simulink model "TTS2_EXT"  (R2024b)
settings: Solver=FixedStepAuto  StartTime=0.0  StopTime=inf  FixedStep=0.01  RelTol=1e-3
model workspace (MAT data in the model file):
  amp_f1 = -100
  amp_f10 = 0.5
  amp_f11 = -0.1
  amp_f12 = 1
  amp_f13 = 0.5
  amp_f14 = -20
  amp_f15 = 0.5
  amp_f16 = 0.5
  amp_f17 = 20
  amp_f18 = -30
  amp_f19 = 0.1
  amp_f2 = -20
  amp_f20 = -20
  amp_f21 = 20
  amp_f3 = -30
  amp_f4 = -30
  amp_f5 = -10
  amp_f51 = -10
  amp_f52 = -30
  amp_f53 = -30
  amp_f54 = 20
  amp_f55 = -100
  amp_f6 = -30
  amp_f7 = -30
  amp_f8 = -30
  amp_f9 = 1
  from_f1 = 570
  from_f10 = 5970
  from_f11 = 6570
  from_f12 = 7170
  from_f13 = 7770
  from_f14 = 8370
  from_f15 = 8970
  from_f16 = 9570
  from_f17 = 10170
  from_f18 = 10770
  from_f19 = 11370
  from_f2 = 1170
  from_f20 = 11970
  from_f21 = 12570
  from_f3 = 1770
  from_f4 = 2370
  from_f5 = 2970
  from_f51 = 13170
  from_f52 = 13770
  from_f53 = 14370
  from_f54 = 14970
  from_f55 = 15570
  from_f6 = 3570
  from_f7 = 4170
  from_f8 = 4770
  from_f9 = 5370
libraries: simulink x52, lab310_library x26, opclib x3
(part 3 of 3)

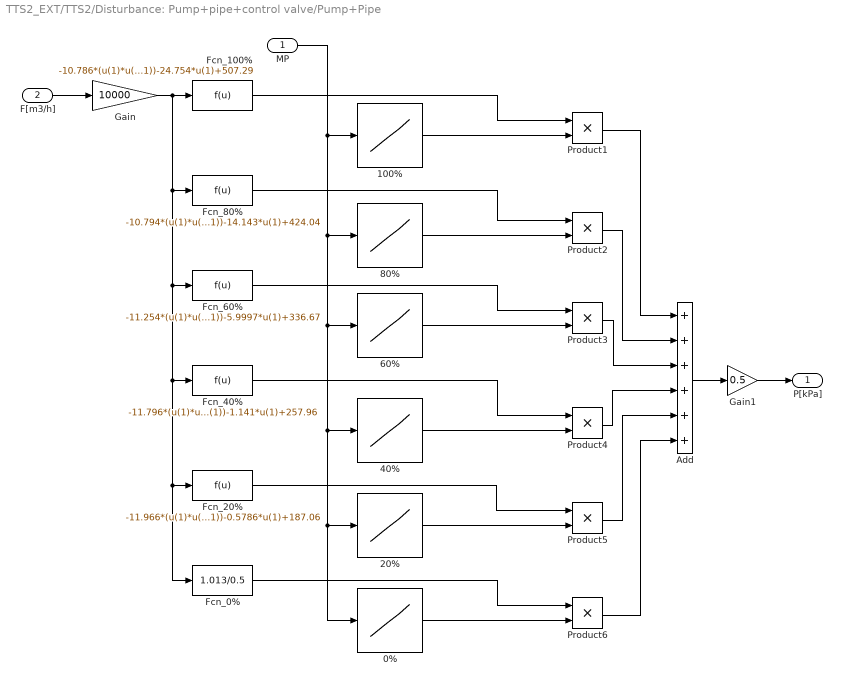
== system TTS2_EXT/TTS2/Disturbance: Pump+pipe+control valve/Pump+Pipe ==
  MP : Inport
  F[m3/h] : Inport  Port=2
  "0% " : Lookup_n-D  NumberOfTableDimensions=1  BreakpointsForDimension1=[0 20 100]  Table=[1 0 0]  InternalRulePriority=Speed  RndMeth=Simplest
  100% : Lookup_n-D  NumberOfTableDimensions=1  BreakpointsForDimension1=[0 80 100]  Table=[0 0 1]  InternalRulePriority=Speed  RndMeth=Simplest
  20% : Lookup_n-D  NumberOfTableDimensions=1  BreakpointsForDimension1=[0 20 40 100]  Table=[0 1 0 0]  InternalRulePriority=Speed  RndMeth=Simplest
  40% : Lookup_n-D  NumberOfTableDimensions=1  BreakpointsForDimension1=[0 20 40 60 100]  Table=[0 0 1 0 0]  InternalRulePriority=Speed  RndMeth=Simplest
  60% : Lookup_n-D  NumberOfTableDimensions=1  BreakpointsForDimension1=[0 40 60 80 100]  Table=[0 0 1 0 0]  InternalRulePriority=Speed  RndMeth=Simplest
  80% : Lookup_n-D  NumberOfTableDimensions=1  BreakpointsForDimension1=[0 60 80 100]  Table=[0 0 1 0]  InternalRulePriority=Speed  RndMeth=Simplest
  Add : Sum  Inputs=6
  Fcn_0% : Fcn  Expr=1.013/0.5
  Fcn_100% : Fcn  Expr=-10.786*(u(1)*u(1))-24.754*u(1)+507.29
  Fcn_20% : Fcn  Expr=-11.966*(u(1)*u(1))-0.5786*u(1)+187.06
  Fcn_40% : Fcn  Expr=-11.796*(u(1)*u(1))-1.141*u(1)+257.96
  Fcn_60% : Fcn  Expr=-11.254*(u(1)*u(1))-5.9997*u(1)+336.67
  Fcn_80% : Fcn  Expr=-10.794*(u(1)*u(1))-14.143*u(1)+424.04
  Gain : Gain  Gain=10000
  Gain1 : Gain  Gain=0.5
  Product{1..6} (6 alike) : Product
  P[kPa] : Outport  VectorParamsAs1DForOutWhenUnconnected=off
  wires:
  F[m3/h]/1 -> Gain/1
  MP/1 -> 80%/1, 40%/1, 20%/1, "0% "/1, 60%/1, 100%/1
  "0% "/1 -> Product6/2
  20%/1 -> Product5/2
  40%/1 -> Product4/2
  60%/1 -> Product3/2
  80%/1 -> Product2/2
  100%/1 -> Product1/2
  Gain/1 -> Fcn_20%/1, Fcn_0%/1, Fcn_40%/1, Fcn_60%/1, Fcn_80%/1, Fcn_100%/1
  Fcn_0%/1 -> Product6/1
  Fcn_20%/1 -> Product5/1
  Fcn_40%/1 -> Product4/1
  Fcn_60%/1 -> Product3/1
  Fcn_80%/1 -> Product2/1
  Fcn_100%/1 -> Product1/1
  Product1/1 -> Add/1
  Product2/1 -> Add/2
  Product3/1 -> Add/3
  Product4/1 -> Add/4
  Product5/1 -> Add/5
  Product6/1 -> Add/6
  Add/1 -> Gain1/1
  Gain1/1 -> P[kPa]/1

== system TTS2_EXT/TTS2/Disturbance: Pump+pipe+control valve/VB ==
  CV[%] : Inport
  P1[kPa] : Inport  Port=2
  P2[kPa] : Inport  Port=3
  Positioner : Subsystem
  Valve : Subsystem
  F[m3/h] : Outport  VectorParamsAs1DForOutWhenUnconnected=off
  wires:
  Valve/1(F[m3/h]) -> F[m3/h]/1
  P1[kPa]/1 -> Valve/2(P1[kPa])
  P2[kPa]/1 -> Valve/3(P2[kPa])
  CV[%]/1 -> Positioner/1(CV[0-100])
  Positioner/1(X[0-1]) -> Valve/1(G[0-1])

== system TTS2_EXT/TTS2/Noise/F1 noise ==
  X : Inport
  Random Number : RandomNumber  Variance=0.006889  Seed=3341  SampleTime=1
  Sum : Sum  Inputs=|++
  X' : Outport  VectorParamsAs1DForOutWhenUnconnected=off
  wires:
  Random Number/1 -> Sum/2
  X/1 -> Sum/1
  Sum/1 -> X'/1

== system TTS2_EXT/TTS2/Noise/F2 noise ==
  X : Inport
  Random Number : RandomNumber  Variance=0.0225  Seed=765756  SampleTime=1
  Sum : Sum  Inputs=|++
  X' : Outport  VectorParamsAs1DForOutWhenUnconnected=off
  wires:
  Random Number/1 -> Sum/2
  X/1 -> Sum/1
  Sum/1 -> X'/1

== system TTS2_EXT/TTS2/Noise/F3 dist ==
  X : Inport
  Random Number : RandomNumber  Variance=0.0225  Seed=756756  SampleTime=1
  Sum : Sum  Inputs=|++
  X' : Outport  VectorParamsAs1DForOutWhenUnconnected=off
  wires:
  Random Number/1 -> Sum/2
  X/1 -> Sum/1
  Sum/1 -> X'/1

== system TTS2_EXT/TTS2/Noise/G noise ==
  X : Inport
  Random Number : RandomNumber  Variance=0.006889  Seed=2312  SampleTime=1
  Sum : Sum  Inputs=|++
  X' : Outport  VectorParamsAs1DForOutWhenUnconnected=off
  wires:
  Random Number/1 -> Sum/2
  X/1 -> Sum/1
  Sum/1 -> X'/1

== system TTS2_EXT/TTS2/Noise/G2 noise ==
  X : Inport
  Random Number : RandomNumber  Variance=0.0225  Seed=75675675  SampleTime=1
  Sum : Sum  Inputs=|++
  X' : Outport  VectorParamsAs1DForOutWhenUnconnected=off
  wires:
  Random Number/1 -> Sum/2
  X/1 -> Sum/1
  Sum/1 -> X'/1

== system TTS2_EXT/TTS2/Noise/L11 noise ==
  X : Inport
  Random Number : RandomNumber  Variance=0.000002777  Seed=4324  SampleTime=1
  Sum : Sum  Inputs=|++
  X' : Outport  VectorParamsAs1DForOutWhenUnconnected=off
  wires:
  Random Number/1 -> Sum/2
  X/1 -> Sum/1
  Sum/1 -> X'/1

== system TTS2_EXT/TTS2/Noise/L12 noise ==
  X : Inport
  Random Number : RandomNumber  Variance=0.00000053777  Seed=432423  SampleTime=1
  Sum : Sum  Inputs=|++
  X' : Outport  VectorParamsAs1DForOutWhenUnconnected=off
  wires:
  Random Number/1 -> Sum/2
  X/1 -> Sum/1
  Sum/1 -> X'/1

== system TTS2_EXT/TTS2/Noise/L21 noise ==
  X : Inport
  Random Number : RandomNumber  Variance=0.000000111111111  Seed=43243423  SampleTime=1
  Sum : Sum  Inputs=|++
  X' : Outport  VectorParamsAs1DForOutWhenUnconnected=off
  wires:
  Random Number/1 -> Sum/2
  X/1 -> Sum/1
  Sum/1 -> X'/1

== system TTS2_EXT/TTS2/Noise/L22 noise ==
  X : Inport
  Random Number : RandomNumber  Variance=0.0000001111111111  Seed=32423  SampleTime=1
  Sum : Sum  Inputs=|++
  X' : Outport  VectorParamsAs1DForOutWhenUnconnected=off
  wires:
  Random Number/1 -> Sum/2
  X/1 -> Sum/1
  Sum/1 -> X'/1

== system TTS2_EXT/TTS2/Noise/L31 noise ==
  X : Inport
  Random Number : RandomNumber  Variance=0.0000017777  Seed=432454  SampleTime=1
  Sum : Sum  Inputs=|++
  X' : Outport  VectorParamsAs1DForOutWhenUnconnected=off
  wires:
  Random Number/1 -> Sum/2
  X/1 -> Sum/1
  Sum/1 -> X'/1

== system TTS2_EXT/TTS2/Noise/L32 noise ==
  X : Inport
  Random Number : RandomNumber  Variance=0.0000006944  Seed=4563565  SampleTime=1
  Sum : Sum  Inputs=|++
  X' : Outport  VectorParamsAs1DForOutWhenUnconnected=off
  wires:
  Random Number/1 -> Sum/2
  X/1 -> Sum/1
  Sum/1 -> X'/1

== system TTS2_EXT/TTS2/Noise/P Dist ==
  X : Inport
  Random Number : RandomNumber  Variance=0.09  Seed=32321  SampleTime=1
  Sum : Sum  Inputs=|++
  X' : Outport  VectorParamsAs1DForOutWhenUnconnected=off
  wires:
  Random Number/1 -> Sum/2
  X/1 -> Sum/1
  Sum/1 -> X'/1

== system TTS2_EXT/TTS2/Noise/dP dist ==
  X : Inport
  Random Number : RandomNumber  Variance=0.09  Seed=756756756  SampleTime=1
  Sum : Sum  Inputs=|++
  X' : Outport  VectorParamsAs1DForOutWhenUnconnected=off
  wires:
  Random Number/1 -> Sum/2
  X/1 -> Sum/1
  Sum/1 -> X'/1

== system TTS2_EXT/TTS2/Noise/f11 fault ==
  X : Inport
  str. : Inport  Port=2
  Add : Sum
  Fcn : Fcn  Expr=u(1)*((u(2)/100)+1)
  Manual Switch : ManualSwitch
  Mux : Mux  Inputs=2
  X' : Outport  VectorParamsAs1DForOutWhenUnconnected=off
  wires:
  Mux/1 -> Fcn/1
  X/1 -> Add/1, Mux/1
  str./1 -> Add/2, Mux/2
  Add/1 -> Manual Switch/1
  Fcn/1 -> Manual Switch/2
  Manual Switch/1 -> X'/1

== system TTS2_EXT/TTS2/Noise/f14 fault ==
  X : Inport
  str. : Inport  Port=2
  Add : Sum
  Fcn : Fcn  Expr=u(1)*((u(2)/100)+1)
  Manual Switch : ManualSwitch  CurrentSetting=0
  Mux : Mux  Inputs=2
  X' : Outport  VectorParamsAs1DForOutWhenUnconnected=off
  wires:
  Mux/1 -> Fcn/1
  X/1 -> Add/1, Mux/1
  str./1 -> Add/2, Mux/2
  Add/1 -> Manual Switch/1
  Fcn/1 -> Manual Switch/2
  Manual Switch/1 -> X'/1

== system TTS2_EXT/TTS2/Noise/f17 fault ==
  X : Inport
  str. : Inport  Port=2
  Add : Sum
  Fcn : Fcn  Expr=u(1)*((u(2)/100)+1)
  Manual Switch : ManualSwitch  CurrentSetting=0
  Mux : Mux  Inputs=2
  X' : Outport  VectorParamsAs1DForOutWhenUnconnected=off
  wires:
  Mux/1 -> Fcn/1
  X/1 -> Add/1, Mux/1
  str./1 -> Add/2, Mux/2
  Add/1 -> Manual Switch/1
  Fcn/1 -> Manual Switch/2
  Manual Switch/1 -> X'/1

== system TTS2_EXT/TTS2/Noise/f18 fault ==
  X : Inport
  str. : Inport  Port=2
  Add : Sum
  Fcn : Fcn  Expr=u(1)*((u(2)/100)+1)
  Manual Switch : ManualSwitch  CurrentSetting=0
  Mux : Mux  Inputs=2
  X' : Outport  VectorParamsAs1DForOutWhenUnconnected=off
  wires:
  Mux/1 -> Fcn/1
  X/1 -> Add/1, Mux/1
  str./1 -> Add/2, Mux/2
  Fcn/1 -> Manual Switch/2
  Manual Switch/1 -> X'/1
  Add/1 -> Manual Switch/1

== system TTS2_EXT/TTS2/Noise/f19 fault ==
  X : Inport
  str. : Inport  Port=2
  Add : Sum
  Fcn : Fcn  Expr=u(1)*((u(2)/100)+1)
  Manual Switch : ManualSwitch
  Mux : Mux  Inputs=2
  X' : Outport  VectorParamsAs1DForOutWhenUnconnected=off
  wires:
  Mux/1 -> Fcn/1
  X/1 -> Add/1, Mux/1
  str./1 -> Add/2, Mux/2
  Add/1 -> Manual Switch/1
  Fcn/1 -> Manual Switch/2
  Manual Switch/1 -> X'/1

== system TTS2_EXT/TTS2/Noise/f20 fault ==
  X : Inport
  str. : Inport  Port=2
  Add : Sum
  Fcn : Fcn  Expr=u(1)*((u(2)/100)+1)
  Manual Switch : ManualSwitch  CurrentSetting=0
  Mux : Mux  Inputs=2
  X' : Outport  VectorParamsAs1DForOutWhenUnconnected=off
  wires:
  Mux/1 -> Fcn/1
  X/1 -> Add/1, Mux/1
  str./1 -> Add/2, Mux/2
  Add/1 -> Manual Switch/1
  Fcn/1 -> Manual Switch/2
  Manual Switch/1 -> X'/1

== system TTS2_EXT/TTS2/Noise/f21 fault ==
  X : Inport
  str. : Inport  Port=2
  Add : Sum
  Fcn : Fcn  Expr=u(1)*((u(2)/100)+1)
  Manual Switch : ManualSwitch  CurrentSetting=0
  Mux : Mux  Inputs=2
  X' : Outport  VectorParamsAs1DForOutWhenUnconnected=off
  wires:
  Mux/1 -> Fcn/1
  X/1 -> Add/1, Mux/1
  str./1 -> Add/2, Mux/2
  Add/1 -> Manual Switch/1
  Fcn/1 -> Manual Switch/2
  Manual Switch/1 -> X'/1

== system TTS2_EXT/TTS2/Noise/f5 fault ==
  X : Inport
  str. : Inport  Port=2
  Add : Sum
  Fcn : Fcn  Expr=u(1)*((u(2)/100)+1)
  Manual Switch : ManualSwitch
  Mux : Mux  Inputs=2
  X' : Outport  VectorParamsAs1DForOutWhenUnconnected=off
  wires:
  Mux/1 -> Fcn/1
  X/1 -> Add/1, Mux/1
  str./1 -> Add/2, Mux/2
  Add/1 -> Manual Switch/1
  Fcn/1 -> Manual Switch/2
  Manual Switch/1 -> X'/1

== system TTS2_EXT/TTS2/Noise/f51 fault ==
  X : Inport
  str. : Inport  Port=2
  Add : Sum
  Fcn : Fcn  Expr=u(1)*((u(2)/100)+1)
  Manual Switch : ManualSwitch
  Mux : Mux  Inputs=2
  X' : Outport  VectorParamsAs1DForOutWhenUnconnected=off
  wires:
  Mux/1 -> Fcn/1
  X/1 -> Add/1, Mux/1
  str./1 -> Add/2, Mux/2
  Add/1 -> Manual Switch/1
  Fcn/1 -> Manual Switch/2
  Manual Switch/1 -> X'/1

== system TTS2_EXT/TTS2/Noise/f52 fault ==
  X : Inport
  str. : Inport  Port=2
  Add : Sum
  Fcn : Fcn  Expr=u(1)*((u(2)/100)+1)
  Manual Switch : ManualSwitch  CurrentSetting=0
  Mux : Mux  Inputs=2
  X' : Outport  VectorParamsAs1DForOutWhenUnconnected=off
  wires:
  Mux/1 -> Fcn/1
  X/1 -> Add/1, Mux/1
  str./1 -> Add/2, Mux/2
  Add/1 -> Manual Switch/1
  Fcn/1 -> Manual Switch/2
  Manual Switch/1 -> X'/1

== system TTS2_EXT/TTS2/Noise/f54 fault ==
  X : Inport
  str. : Inport  Port=2
  Add : Sum
  Fcn : Fcn  Expr=u(1)*((u(2)/100)+1)
  Manual Switch : ManualSwitch  CurrentSetting=0
  Mux : Mux  Inputs=2
  X' : Outport  VectorParamsAs1DForOutWhenUnconnected=off
  wires:
  Mux/1 -> Fcn/1
  X/1 -> Add/1, Mux/1
  str./1 -> Add/2, Mux/2
  Add/1 -> Manual Switch/1
  Fcn/1 -> Manual Switch/2
  Manual Switch/1 -> X'/1

== system TTS2_EXT/TTS2/Noise/f7 fault ==
  X : Inport
  str. : Inport  Port=2
  Add : Sum
  Fcn : Fcn  Expr=u(1)*((u(2)/100)+1)
  Manual Switch : ManualSwitch  CurrentSetting=0
  Mux : Mux  Inputs=2
  X' : Outport  VectorParamsAs1DForOutWhenUnconnected=off
  wires:
  Mux/1 -> Fcn/1
  X/1 -> Add/1, Mux/1
  str./1 -> Add/2, Mux/2
  Add/1 -> Manual Switch/1
  Fcn/1 -> Manual Switch/2
  Manual Switch/1 -> X'/1

== system TTS2_EXT/TTS2/Noise/f8 fault ==
  X : Inport
  str. : Inport  Port=2
  Add : Sum
  Fcn : Fcn  Expr=u(1)*((u(2)/100)+1)
  Manual Switch : ManualSwitch  CurrentSetting=0
  Mux : Mux  Inputs=2
  X' : Outport  VectorParamsAs1DForOutWhenUnconnected=off
  wires:
  Mux/1 -> Fcn/1
  X/1 -> Add/1, Mux/1
  str./1 -> Add/2, Mux/2
  Add/1 -> Manual Switch/1
  Fcn/1 -> Manual Switch/2
  Manual Switch/1 -> X'/1

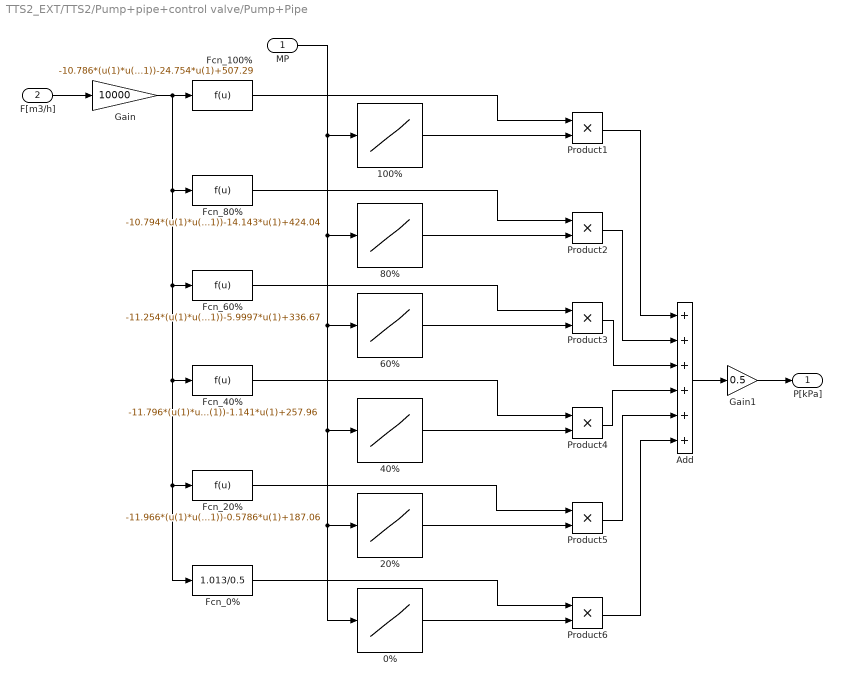
== system TTS2_EXT/TTS2/Pump+pipe+control valve/Pump+Pipe ==
  MP : Inport
  F[m3/h] : Inport  Port=2
  "0% " : Lookup_n-D  NumberOfTableDimensions=1  BreakpointsForDimension1=[0 20 100]  Table=[1 0 0]  InternalRulePriority=Speed  RndMeth=Simplest
  100% : Lookup_n-D  NumberOfTableDimensions=1  BreakpointsForDimension1=[0 80 100]  Table=[0 0 1]  InternalRulePriority=Speed  RndMeth=Simplest
  20% : Lookup_n-D  NumberOfTableDimensions=1  BreakpointsForDimension1=[0 20 40 100]  Table=[0 1 0 0]  InternalRulePriority=Speed  RndMeth=Simplest
  40% : Lookup_n-D  NumberOfTableDimensions=1  BreakpointsForDimension1=[0 20 40 60 100]  Table=[0 0 1 0 0]  InternalRulePriority=Speed  RndMeth=Simplest
  60% : Lookup_n-D  NumberOfTableDimensions=1  BreakpointsForDimension1=[0 40 60 80 100]  Table=[0 0 1 0 0]  InternalRulePriority=Speed  RndMeth=Simplest
  80% : Lookup_n-D  NumberOfTableDimensions=1  BreakpointsForDimension1=[0 60 80 100]  Table=[0 0 1 0]  InternalRulePriority=Speed  RndMeth=Simplest
  Add : Sum  Inputs=6
  Fcn_0% : Fcn  Expr=1.013/0.5
  Fcn_100% : Fcn  Expr=-10.786*(u(1)*u(1))-24.754*u(1)+507.29
  Fcn_20% : Fcn  Expr=-11.966*(u(1)*u(1))-0.5786*u(1)+187.06
  Fcn_40% : Fcn  Expr=-11.796*(u(1)*u(1))-1.141*u(1)+257.96
  Fcn_60% : Fcn  Expr=-11.254*(u(1)*u(1))-5.9997*u(1)+336.67
  Fcn_80% : Fcn  Expr=-10.794*(u(1)*u(1))-14.143*u(1)+424.04
  Gain : Gain  Gain=10000
  Gain1 : Gain  Gain=0.5
  Product{1..6} (6 alike) : Product
  P[kPa] : Outport  VectorParamsAs1DForOutWhenUnconnected=off
  wires:
  F[m3/h]/1 -> Gain/1
  MP/1 -> 80%/1, 40%/1, 20%/1, "0% "/1, 60%/1, 100%/1
  "0% "/1 -> Product6/2
  20%/1 -> Product5/2
  40%/1 -> Product4/2
  60%/1 -> Product3/2
  80%/1 -> Product2/2
  100%/1 -> Product1/2
  Gain/1 -> Fcn_20%/1, Fcn_0%/1, Fcn_40%/1, Fcn_60%/1, Fcn_80%/1, Fcn_100%/1
  Fcn_0%/1 -> Product6/1
  Fcn_20%/1 -> Product5/1
  Fcn_40%/1 -> Product4/1
  Fcn_60%/1 -> Product3/1
  Fcn_80%/1 -> Product2/1
  Fcn_100%/1 -> Product1/1
  Product1/1 -> Add/1
  Product2/1 -> Add/2
  Product3/1 -> Add/3
  Product4/1 -> Add/4
  Product5/1 -> Add/5
  Product6/1 -> Add/6
  Add/1 -> Gain1/1
  Gain1/1 -> P[kPa]/1

== system TTS2_EXT/TTS2/Pump+pipe+control valve/V1 ==
  CV[%] : Inport
  P1[kPa] : Inport  Port=2
  P2[kPa] : Inport  Port=3
  f04 : Inport  Port=4
  f06 : Inport  Port=5
  Gain2 : Gain  Gain=100
  Positioner : Subsystem
  Saturation : Saturate  UpperLimit=1  LowerLimit=0
  Valve : Subsystem
  f4 fault : Subsystem
  f6 fault : Subsystem
  X[%] : Outport  VectorParamsAs1DForOutWhenUnconnected=off
  F[m3/s] : Outport  Port=2  VectorParamsAs1DForOutWhenUnconnected=off
  dP[kPa] : Outport  Port=3  VectorParamsAs1DForOutWhenUnconnected=off
  wires:
  Valve/1(dP[kPa]) -> dP[kPa]/1
  Valve/2(F[m3/s]) -> F[m3/s]/1
  P1[kPa]/1 -> Valve/2(P1[kPa])
  P2[kPa]/1 -> Valve/3(P2[kPa])
  f06/1 -> f6 fault/2(str.)
  f6 fault/1(Xf) -> Saturation/1
  f4 fault/1(Xf) -> Positioner/1(CV[0-100])
  f04/1 -> f4 fault/2(str.)
  Positioner/1(X[0-1]) -> f6 fault/1(X), Gain2/1
  CV[%]/1 -> f4 fault/1(X)
  Gain2/1 -> X[%]/1
  Saturation/1 -> Valve/1(G[0-1])

== system TTS2_EXT/TTS2/Pump+pipe+control valve/V2 ==
  CV[%] : Inport
  P1[kPa] : Inport  Port=2
  P2[kPa] : Inport  Port=3
  f53 : Inport  Port=4
  Gain2 : Gain  Gain=100
  Positioner : Subsystem
  Saturation : Saturate  UpperLimit=1  LowerLimit=0
  Valve : Subsystem
  f53 fault : Subsystem
  X[%] : Outport  VectorParamsAs1DForOutWhenUnconnected=off
  F[m3/s] : Outport  Port=2  VectorParamsAs1DForOutWhenUnconnected=off
  dP[kPa] : Outport  Port=3  VectorParamsAs1DForOutWhenUnconnected=off
  wires:
  Valve/1(dP[kPa]) -> dP[kPa]/1
  Valve/2(F[m3/s]) -> F[m3/s]/1
  P1[kPa]/1 -> Valve/2(P1[kPa])
  P2[kPa]/1 -> Valve/3(P2[kPa])
  f53/1 -> f53 fault/2(str.)
  f53 fault/1(Xf) -> Saturation/1
  CV[%]/1 -> Positioner/1(CV[0-100])
  Positioner/1(X[0-1]) -> f53 fault/1(X), Gain2/1
  Gain2/1 -> X[%]/1
  Saturation/1 -> Valve/1(G[0-1])

== system TTS2_EXT/TTS2/Pump+pipe+control valve/f1 fault ==
  X : Inport
  str. : Inport  Port=2
  Add : Sum
  Fcn1 : Fcn  Expr=u(1)*((u(2)/100)+1)
  Manual Switch : ManualSwitch  CurrentSetting=0
  Mux1 : Mux  Inputs=2
  Xf : Outport  VectorParamsAs1DForOutWhenUnconnected=off
  wires:
  Mux1/1 -> Fcn1/1
  X/1 -> Add/1, Mux1/1
  str./1 -> Add/2, Mux1/2
  Add/1 -> Manual Switch/1
  Fcn1/1 -> Manual Switch/2
  Manual Switch/1 -> Xf/1

== system TTS2_EXT/TTS2/Pump+pipe+control valve/f2 fault ==
  X : Inport
  str. : Inport  Port=2
  Add : Sum
  Fcn : Fcn  Expr=u(1)*((u(2)/100)+1)
  Manual Switch : ManualSwitch  CurrentSetting=0
  Mux : Mux  Inputs=2
  Xf : Outport  VectorParamsAs1DForOutWhenUnconnected=off
  wires:
  Mux/1 -> Fcn/1
  X/1 -> Add/1, Mux/1
  str./1 -> Add/2, Mux/2
  Add/1 -> Manual Switch/1
  Fcn/1 -> Manual Switch/2
  Manual Switch/1 -> Xf/1

== system TTS2_EXT/TTS2/Tanks/Pipe 1-2 ==
  h1 : Inport
  k : Inport  Port=2
  h2 : Inport  Port=3
  Fcn : Fcn  Expr=sqrt(abs(u(1)*2*9.81))
  Product : Product  Inputs=3
  Sign : Signum
  Subtract : Sum  Inputs=+-
  F : Outport  VectorParamsAs1DForOutWhenUnconnected=off
  wires:
  h1/1 -> Subtract/1
  h2/1 -> Subtract/2
  Subtract/1 -> Sign/1, Fcn/1
  Fcn/1 -> Product/1
  Sign/1 -> Product/2
  k/1 -> Product/3
  Product/1 -> F/1

== system TTS2_EXT/TTS2/Tanks/Pipe 2-3 ==
  h1 : Inport
  k : Inport  Port=2
  h2 : Inport  Port=3
  Fcn : Fcn  Expr=sqrt(abs(u(1)*2*9.81))
  Product : Product  Inputs=3
  Sign : Signum
  Subtract : Sum  Inputs=+-
  F : Outport  VectorParamsAs1DForOutWhenUnconnected=off
  wires:
  h1/1 -> Subtract/1
  h2/1 -> Subtract/2
  Subtract/1 -> Sign/1, Fcn/1
  Fcn/1 -> Product/1
  Sign/1 -> Product/2
  k/1 -> Product/3
  Product/1 -> F/1

== system TTS2_EXT/TTS2/Tanks/Pipe 3-0 ==
  h1 : Inport
  k : Inport  Port=2
  h2 : Inport  Port=3
  Fcn : Fcn  Expr=sqrt(abs(u(1)*2*9.81))
  Product : Product  Inputs=3
  Sign : Signum
  Subtract : Sum  Inputs=+-
  F : Outport  VectorParamsAs1DForOutWhenUnconnected=off
  wires:
  h1/1 -> Subtract/1
  h2/1 -> Subtract/2
  Subtract/1 -> Sign/1, Fcn/1
  Fcn/1 -> Product/1
  Sign/1 -> Product/2
  k/1 -> Product/3
  Product/1 -> F/1

== system TTS2_EXT/TTS2/Tanks/Tank 1  ==
  F in : Inport
  F1 : Inport  Port=2
  A : Inport  Port=3
  kw : Inport  Port=4
  F2 : Inport  Port=5
  Divide : Product  Inputs=*/
  Gain : Gain  Gain=19.62
  Integrator : Integrator  LimitOutput=on  UpperSaturationLimit=1  LowerSaturationLimit=0
  Sqrt : Sqrt
  Subtract : Sum  Inputs=+++-
  multiply : Product  Inputs=**
  L : Outport  VectorParamsAs1DForOutWhenUnconnected=off
  wires:
  F in/1 -> Subtract/1
  F1/1 -> Subtract/2
  F2/1 -> Subtract/3
  Subtract/1 -> Divide/1
  A/1 -> Divide/2
  Divide/1 -> Integrator/1
  Integrator/1 -> Gain/1, L/1
  kw/1 -> multiply/1
  Sqrt/1 -> multiply/2
  Gain/1 -> Sqrt/1
  multiply/1 -> Subtract/4

== system TTS2_EXT/TTS2/Tanks/Tank 2 ==
  F in : Inport
  F1 : Inport  Port=2
  A : Inport  Port=3
  kw : Inport  Port=4
  F2 : Inport  Port=5
  Divide : Product  Inputs=*/
  Gain : Gain  Gain=19.62
  Integrator : Integrator  LimitOutput=on  UpperSaturationLimit=1  LowerSaturationLimit=0
  Sqrt : Sqrt
  Subtract : Sum  Inputs=+++-
  multiply : Product  Inputs=**
  L : Outport  VectorParamsAs1DForOutWhenUnconnected=off
  wires:
  F in/1 -> Subtract/1
  F1/1 -> Subtract/2
  F2/1 -> Subtract/3
  Subtract/1 -> Divide/1
  A/1 -> Divide/2
  Divide/1 -> Integrator/1
  Integrator/1 -> Gain/1, L/1
  kw/1 -> multiply/1
  Sqrt/1 -> multiply/2
  Gain/1 -> Sqrt/1
  multiply/1 -> Subtract/4

== system TTS2_EXT/TTS2/Tanks/Tank 3 ==
  F in : Inport
  F1 : Inport  Port=2
  A : Inport  Port=3
  kw : Inport  Port=4
  F2 : Inport  Port=5
  Divide : Product  Inputs=*/
  Gain : Gain  Gain=19.62
  Integrator : Integrator  LimitOutput=on  UpperSaturationLimit=1  LowerSaturationLimit=0
  Sqrt : Sqrt
  Subtract : Sum  Inputs=+++-
  multiply : Product  Inputs=**
  L : Outport  VectorParamsAs1DForOutWhenUnconnected=off
  wires:
  F in/1 -> Subtract/1
  F1/1 -> Subtract/2
  F2/1 -> Subtract/3
  Subtract/1 -> Divide/1
  A/1 -> Divide/2
  Divide/1 -> Integrator/1
  Integrator/1 -> Gain/1, L/1
  kw/1 -> multiply/1
  Sqrt/1 -> multiply/2
  Gain/1 -> Sqrt/1
  multiply/1 -> Subtract/4

== system TTS2_EXT/TTS2/Tanks/f55 fault ==
  X : Inport
  str. : Inport  Port=2
  Logical Operator : Logic  Operator=NOT  AllPortsSameDT=off  OutDataTypeStr=boolean
  Switch2 : Switch  Criteria=u2 > Threshold  SaturateOnIntegerOverflow=off  InputSameDT=off
  X' : Outport  VectorParamsAs1DForOutWhenUnconnected=off
  wires:
  Switch2/1 -> X'/1
  str./1 -> Switch2/2
  X/1 -> Switch2/3, Logical Operator/1
  Logical Operator/1 -> Switch2/1

== system TTS2_EXT/Faults/f-control1/calc_f1/Subsystem ==
  w : Inport
  Product1 : Product
  Step2 : Step  Time=t  SampleTime=0
  w_sim : Outport
  wires:
  w/1 -> Product1/1
  Product1/1 -> w_sim/1
  Step2/1 -> Product1/2

== system TTS2_EXT/Faults/f-control1/calc_f10/Subsystem ==
  IncipF : Inport
  w : Inport  Port=2
  Product1 : Product
  RAMP1 : simulink/Sources/Ramp  slope=1/st  start=t  InitialOutput=0
  Saturation1 : Saturate  UpperLimit=1  LowerLimit=0
  Step2 : Step  Time=t  SampleTime=0
  Switch:kind1 : Switch  Criteria=u2 > Threshold  Threshold=0.5  SaturateOnIntegerOverflow=off  InputSameDT=off
  w_sim : Outport
  wires:
  RAMP1/1 -> Saturation1/1
  Saturation1/1 -> Switch:kind1/1
  Switch:kind1/1 -> Product1/2
  w/1 -> Product1/1
  Step2/1 -> Switch:kind1/3
  Product1/1 -> w_sim/1
  IncipF/1 -> Switch:kind1/2

== system TTS2_EXT/Faults/f-control1/calc_f11/Subsystem ==
  IncipF : Inport
  w : Inport  Port=2
  Product1 : Product
  RAMP1 : simulink/Sources/Ramp  slope=1/st  start=t  InitialOutput=0
  Saturation1 : Saturate  UpperLimit=1  LowerLimit=0
  Step2 : Step  Time=t  SampleTime=0
  Switch:kind1 : Switch  Criteria=u2 > Threshold  Threshold=0.5  SaturateOnIntegerOverflow=off  InputSameDT=off
  w_sim : Outport
  wires:
  RAMP1/1 -> Saturation1/1
  Saturation1/1 -> Switch:kind1/1
  Switch:kind1/1 -> Product1/2
  w/1 -> Product1/1
  Step2/1 -> Switch:kind1/3
  Product1/1 -> w_sim/1
  IncipF/1 -> Switch:kind1/2

== system TTS2_EXT/Faults/f-control1/calc_f12/Subsystem ==
  IncipF : Inport
  w : Inport  Port=2
  Product1 : Product
  RAMP1 : simulink/Sources/Ramp  slope=1/st  start=t  InitialOutput=0
  Saturation1 : Saturate  UpperLimit=1  LowerLimit=0
  Step2 : Step  Time=t  SampleTime=0
  Switch:kind1 : Switch  Criteria=u2 > Threshold  Threshold=0.5  SaturateOnIntegerOverflow=off  InputSameDT=off
  w_sim : Outport
  wires:
  RAMP1/1 -> Saturation1/1
  Saturation1/1 -> Switch:kind1/1
  Switch:kind1/1 -> Product1/2
  w/1 -> Product1/1
  Step2/1 -> Switch:kind1/3
  Product1/1 -> w_sim/1
  IncipF/1 -> Switch:kind1/2

== system TTS2_EXT/Faults/f-control1/calc_f13/Subsystem ==
  IncipF : Inport
  w : Inport  Port=2
  Product1 : Product
  RAMP1 : simulink/Sources/Ramp  slope=1/st  start=t  InitialOutput=0
  Saturation1 : Saturate  UpperLimit=1  LowerLimit=0
  Step2 : Step  Time=t  SampleTime=0
  Switch:kind1 : Switch  Criteria=u2 > Threshold  Threshold=0.5  SaturateOnIntegerOverflow=off  InputSameDT=off
  w_sim : Outport
  wires:
  RAMP1/1 -> Saturation1/1
  Saturation1/1 -> Switch:kind1/1
  Switch:kind1/1 -> Product1/2
  w/1 -> Product1/1
  Step2/1 -> Switch:kind1/3
  Product1/1 -> w_sim/1
  IncipF/1 -> Switch:kind1/2

== system TTS2_EXT/Faults/f-control1/calc_f14/Subsystem ==
  IncipF : Inport
  w : Inport  Port=2
  Product1 : Product
  RAMP1 : simulink/Sources/Ramp  slope=1/st  start=t  InitialOutput=0
  Saturation1 : Saturate  UpperLimit=1  LowerLimit=0
  Step2 : Step  Time=t  SampleTime=0
  Switch:kind1 : Switch  Criteria=u2 > Threshold  Threshold=0.5  SaturateOnIntegerOverflow=off  InputSameDT=off
  w_sim : Outport
  wires:
  RAMP1/1 -> Saturation1/1
  Saturation1/1 -> Switch:kind1/1
  Switch:kind1/1 -> Product1/2
  w/1 -> Product1/1
  Step2/1 -> Switch:kind1/3
  Product1/1 -> w_sim/1
  IncipF/1 -> Switch:kind1/2

== system TTS2_EXT/Faults/f-control1/calc_f15/Subsystem ==
  IncipF : Inport
  w : Inport  Port=2
  Product1 : Product
  RAMP1 : simulink/Sources/Ramp  slope=1/st  start=t  InitialOutput=0
  Saturation1 : Saturate  UpperLimit=1  LowerLimit=0
  Step2 : Step  Time=t  SampleTime=0
  Switch:kind1 : Switch  Criteria=u2 > Threshold  Threshold=0.5  SaturateOnIntegerOverflow=off  InputSameDT=off
  w_sim : Outport
  wires:
  RAMP1/1 -> Saturation1/1
  Saturation1/1 -> Switch:kind1/1
  Switch:kind1/1 -> Product1/2
  w/1 -> Product1/1
  Step2/1 -> Switch:kind1/3
  Product1/1 -> w_sim/1
  IncipF/1 -> Switch:kind1/2

== system TTS2_EXT/Faults/f-control1/calc_f16/Subsystem ==
  IncipF : Inport
  w : Inport  Port=2
  Product1 : Product
  RAMP1 : simulink/Sources/Ramp  slope=1/st  start=t  InitialOutput=0
  Saturation1 : Saturate  UpperLimit=1  LowerLimit=0
  Step2 : Step  Time=t  SampleTime=0
  Switch:kind1 : Switch  Criteria=u2 > Threshold  Threshold=0.5  SaturateOnIntegerOverflow=off  InputSameDT=off
  w_sim : Outport
  wires:
  RAMP1/1 -> Saturation1/1
  Saturation1/1 -> Switch:kind1/1
  Switch:kind1/1 -> Product1/2
  w/1 -> Product1/1
  Step2/1 -> Switch:kind1/3
  Product1/1 -> w_sim/1
  IncipF/1 -> Switch:kind1/2

== system TTS2_EXT/Faults/f-control1/calc_f17/Subsystem ==
  IncipF : Inport
  w : Inport  Port=2
  Product1 : Product
  RAMP1 : simulink/Sources/Ramp  slope=1/st  start=t  InitialOutput=0
  Saturation1 : Saturate  UpperLimit=1  LowerLimit=0
  Step2 : Step  Time=t  SampleTime=0
  Switch:kind1 : Switch  Criteria=u2 > Threshold  Threshold=0.5  SaturateOnIntegerOverflow=off  InputSameDT=off
  w_sim : Outport
  wires:
  RAMP1/1 -> Saturation1/1
  Saturation1/1 -> Switch:kind1/1
  Switch:kind1/1 -> Product1/2
  w/1 -> Product1/1
  Step2/1 -> Switch:kind1/3
  Product1/1 -> w_sim/1
  IncipF/1 -> Switch:kind1/2

== system TTS2_EXT/Faults/f-control1/calc_f18/Subsystem ==
  IncipF : Inport
  w : Inport  Port=2
  Product1 : Product
  RAMP1 : simulink/Sources/Ramp  slope=1/st  start=t  InitialOutput=0
  Saturation1 : Saturate  UpperLimit=1  LowerLimit=0
  Step2 : Step  Time=t  SampleTime=0
  Switch:kind1 : Switch  Criteria=u2 > Threshold  Threshold=0.5  SaturateOnIntegerOverflow=off  InputSameDT=off
  w_sim : Outport
  wires:
  RAMP1/1 -> Saturation1/1
  Saturation1/1 -> Switch:kind1/1
  Switch:kind1/1 -> Product1/2
  w/1 -> Product1/1
  Step2/1 -> Switch:kind1/3
  Product1/1 -> w_sim/1
  IncipF/1 -> Switch:kind1/2

== system TTS2_EXT/Faults/f-control1/calc_f19/Subsystem ==
  IncipF : Inport
  w : Inport  Port=2
  Product1 : Product
  RAMP1 : simulink/Sources/Ramp  slope=1/st  start=t  InitialOutput=0
  Saturation1 : Saturate  UpperLimit=1  LowerLimit=0
  Step2 : Step  Time=t  SampleTime=0
  Switch:kind1 : Switch  Criteria=u2 > Threshold  Threshold=0.5  SaturateOnIntegerOverflow=off  InputSameDT=off
  w_sim : Outport
  wires:
  RAMP1/1 -> Saturation1/1
  Saturation1/1 -> Switch:kind1/1
  Switch:kind1/1 -> Product1/2
  w/1 -> Product1/1
  Step2/1 -> Switch:kind1/3
  Product1/1 -> w_sim/1
  IncipF/1 -> Switch:kind1/2

== system TTS2_EXT/Faults/f-control1/calc_f2/Subsystem ==
  IncipF : Inport
  w : Inport  Port=2
  Product1 : Product
  RAMP1 : simulink/Sources/Ramp  slope=1/st  start=t  InitialOutput=0
  Saturation1 : Saturate  UpperLimit=1  LowerLimit=0
  Step2 : Step  Time=t  SampleTime=0
  Switch:kind1 : Switch  Criteria=u2 > Threshold  Threshold=0.5  SaturateOnIntegerOverflow=off  InputSameDT=off
  w_sim : Outport
  wires:
  RAMP1/1 -> Saturation1/1
  Saturation1/1 -> Switch:kind1/1
  Switch:kind1/1 -> Product1/2
  w/1 -> Product1/1
  Step2/1 -> Switch:kind1/3
  Product1/1 -> w_sim/1
  IncipF/1 -> Switch:kind1/2

== system TTS2_EXT/Faults/f-control1/calc_f20/Subsystem ==
  IncipF : Inport
  w : Inport  Port=2
  Product1 : Product
  RAMP1 : simulink/Sources/Ramp  slope=1/st  start=t  InitialOutput=0
  Saturation1 : Saturate  UpperLimit=1  LowerLimit=0
  Step2 : Step  Time=t  SampleTime=0
  Switch:kind1 : Switch  Criteria=u2 > Threshold  Threshold=0.5  SaturateOnIntegerOverflow=off  InputSameDT=off
  w_sim : Outport
  wires:
  RAMP1/1 -> Saturation1/1
  Saturation1/1 -> Switch:kind1/1
  Switch:kind1/1 -> Product1/2
  w/1 -> Product1/1
  Step2/1 -> Switch:kind1/3
  Product1/1 -> w_sim/1
  IncipF/1 -> Switch:kind1/2

== system TTS2_EXT/Faults/f-control1/calc_f21/Subsystem ==
  IncipF : Inport
  w : Inport  Port=2
  Product1 : Product
  RAMP1 : simulink/Sources/Ramp  slope=1/st  start=t  InitialOutput=0
  Saturation1 : Saturate  UpperLimit=1  LowerLimit=0
  Step2 : Step  Time=t  SampleTime=0
  Switch:kind1 : Switch  Criteria=u2 > Threshold  Threshold=0.5  SaturateOnIntegerOverflow=off  InputSameDT=off
  w_sim : Outport
  wires:
  RAMP1/1 -> Saturation1/1
  Saturation1/1 -> Switch:kind1/1
  Switch:kind1/1 -> Product1/2
  w/1 -> Product1/1
  Step2/1 -> Switch:kind1/3
  Product1/1 -> w_sim/1
  IncipF/1 -> Switch:kind1/2

== system TTS2_EXT/Faults/f-control1/calc_f22/Subsystem ==
  IncipF : Inport
  w : Inport  Port=2
  Product1 : Product
  RAMP1 : simulink/Sources/Ramp  slope=1/st  start=t  InitialOutput=0
  Saturation1 : Saturate  UpperLimit=1  LowerLimit=0
  Step2 : Step  Time=t  SampleTime=0
  Switch:kind1 : Switch  Criteria=u2 > Threshold  Threshold=0.5  SaturateOnIntegerOverflow=off  InputSameDT=off
  w_sim : Outport
  wires:
  RAMP1/1 -> Saturation1/1
  Saturation1/1 -> Switch:kind1/1
  Switch:kind1/1 -> Product1/2
  w/1 -> Product1/1
  Step2/1 -> Switch:kind1/3
  Product1/1 -> w_sim/1
  IncipF/1 -> Switch:kind1/2

== system TTS2_EXT/Faults/f-control1/calc_f4/Subsystem ==
  IncipF : Inport
  w : Inport  Port=2
  Product1 : Product
  RAMP1 : simulink/Sources/Ramp  slope=1/st  start=t  InitialOutput=0
  Saturation1 : Saturate  UpperLimit=1  LowerLimit=0
  Step2 : Step  Time=t  SampleTime=0
  Switch:kind1 : Switch  Criteria=u2 > Threshold  Threshold=0.5  SaturateOnIntegerOverflow=off  InputSameDT=off
  w_sim : Outport
  wires:
  RAMP1/1 -> Saturation1/1
  Saturation1/1 -> Switch:kind1/1
  Switch:kind1/1 -> Product1/2
  w/1 -> Product1/1
  Step2/1 -> Switch:kind1/3
  Product1/1 -> w_sim/1
  IncipF/1 -> Switch:kind1/2

== system TTS2_EXT/Faults/f-control1/calc_f5/Subsystem ==
  IncipF : Inport
  w : Inport  Port=2
  Product1 : Product
  RAMP1 : simulink/Sources/Ramp  slope=1/st  start=t  InitialOutput=0
  Saturation1 : Saturate  UpperLimit=1  LowerLimit=0
  Step2 : Step  Time=t  SampleTime=0
  Switch:kind1 : Switch  Criteria=u2 > Threshold  Threshold=0.5  SaturateOnIntegerOverflow=off  InputSameDT=off
  w_sim : Outport
  wires:
  RAMP1/1 -> Saturation1/1
  Saturation1/1 -> Switch:kind1/1
  Switch:kind1/1 -> Product1/2
  w/1 -> Product1/1
  Step2/1 -> Switch:kind1/3
  Product1/1 -> w_sim/1
  IncipF/1 -> Switch:kind1/2

== system TTS2_EXT/Faults/f-control1/calc_f51/Subsystem ==
  IncipF : Inport
  w : Inport  Port=2
  Product1 : Product
  RAMP1 : simulink/Sources/Ramp  slope=1/st  start=t  InitialOutput=0
  Saturation1 : Saturate  UpperLimit=1  LowerLimit=0
  Step2 : Step  Time=t  SampleTime=0
  Switch:kind1 : Switch  Criteria=u2 > Threshold  Threshold=0.5  SaturateOnIntegerOverflow=off  InputSameDT=off
  w_sim : Outport
  wires:
  RAMP1/1 -> Saturation1/1
  Saturation1/1 -> Switch:kind1/1
  Switch:kind1/1 -> Product1/2
  w/1 -> Product1/1
  Step2/1 -> Switch:kind1/3
  Product1/1 -> w_sim/1
  IncipF/1 -> Switch:kind1/2

== system TTS2_EXT/Faults/f-control1/calc_f52/Subsystem ==
  IncipF : Inport
  w : Inport  Port=2
  Product1 : Product
  RAMP1 : simulink/Sources/Ramp  slope=1/st  start=t  InitialOutput=0
  Saturation1 : Saturate  UpperLimit=1  LowerLimit=0
  Step2 : Step  Time=t  SampleTime=0
  Switch:kind1 : Switch  Criteria=u2 > Threshold  Threshold=0.5  SaturateOnIntegerOverflow=off  InputSameDT=off
  w_sim : Outport
  wires:
  RAMP1/1 -> Saturation1/1
  Saturation1/1 -> Switch:kind1/1
  Switch:kind1/1 -> Product1/2
  w/1 -> Product1/1
  Step2/1 -> Switch:kind1/3
  Product1/1 -> w_sim/1
  IncipF/1 -> Switch:kind1/2

== system TTS2_EXT/Faults/f-control1/calc_f53/Subsystem ==
  IncipF : Inport
  w : Inport  Port=2
  Product1 : Product
  RAMP1 : simulink/Sources/Ramp  slope=1/st  start=t  InitialOutput=0
  Saturation1 : Saturate  UpperLimit=1  LowerLimit=0
  Step2 : Step  Time=t  SampleTime=0
  Switch:kind1 : Switch  Criteria=u2 > Threshold  Threshold=0.5  SaturateOnIntegerOverflow=off  InputSameDT=off
  w_sim : Outport
  wires:
  RAMP1/1 -> Saturation1/1
  Saturation1/1 -> Switch:kind1/1
  Switch:kind1/1 -> Product1/2
  w/1 -> Product1/1
  Step2/1 -> Switch:kind1/3
  Product1/1 -> w_sim/1
  IncipF/1 -> Switch:kind1/2

== system TTS2_EXT/Faults/f-control1/calc_f54/Subsystem ==
  IncipF : Inport
  w : Inport  Port=2
  Product1 : Product
  RAMP1 : simulink/Sources/Ramp  slope=1/st  start=t  InitialOutput=0
  Saturation1 : Saturate  UpperLimit=1  LowerLimit=0
  Step2 : Step  Time=t  SampleTime=0
  Switch:kind1 : Switch  Criteria=u2 > Threshold  Threshold=0.5  SaturateOnIntegerOverflow=off  InputSameDT=off
  w_sim : Outport
  wires:
  RAMP1/1 -> Saturation1/1
  Saturation1/1 -> Switch:kind1/1
  Switch:kind1/1 -> Product1/2
  w/1 -> Product1/1
  Step2/1 -> Switch:kind1/3
  Product1/1 -> w_sim/1
  IncipF/1 -> Switch:kind1/2

== system TTS2_EXT/Faults/f-control1/calc_f55/Subsystem ==
  w : Inport
  Product1 : Product
  Step2 : Step  Time=t  SampleTime=0
  w_sim : Outport
  wires:
  w/1 -> Product1/1
  Product1/1 -> w_sim/1
  Step2/1 -> Product1/2

== system TTS2_EXT/Faults/f-control1/calc_f6/Subsystem ==
  IncipF : Inport
  w : Inport  Port=2
  Product1 : Product
  RAMP1 : simulink/Sources/Ramp  slope=1/st  start=t  InitialOutput=0
  Saturation1 : Saturate  UpperLimit=1  LowerLimit=0
  Step2 : Step  Time=t  SampleTime=0
  Switch:kind1 : Switch  Criteria=u2 > Threshold  Threshold=0.5  SaturateOnIntegerOverflow=off  InputSameDT=off
  w_sim : Outport
  wires:
  RAMP1/1 -> Saturation1/1
  Saturation1/1 -> Switch:kind1/1
  Switch:kind1/1 -> Product1/2
  w/1 -> Product1/1
  Step2/1 -> Switch:kind1/3
  Product1/1 -> w_sim/1
  IncipF/1 -> Switch:kind1/2

== system TTS2_EXT/Faults/f-control1/calc_f7/Subsystem ==
  IncipF : Inport
  w : Inport  Port=2
  Product1 : Product
  RAMP1 : simulink/Sources/Ramp  slope=1/st  start=t  InitialOutput=0
  Saturation1 : Saturate  UpperLimit=1  LowerLimit=0
  Step2 : Step  Time=t  SampleTime=0
  Switch:kind1 : Switch  Criteria=u2 > Threshold  Threshold=0.5  SaturateOnIntegerOverflow=off  InputSameDT=off
  w_sim : Outport
  wires:
  RAMP1/1 -> Saturation1/1
  Saturation1/1 -> Switch:kind1/1
  Switch:kind1/1 -> Product1/2
  w/1 -> Product1/1
  Step2/1 -> Switch:kind1/3
  Product1/1 -> w_sim/1
  IncipF/1 -> Switch:kind1/2

== system TTS2_EXT/Faults/f-control1/calc_f8/Subsystem ==
  IncipF : Inport
  w : Inport  Port=2
  Product1 : Product
  RAMP1 : simulink/Sources/Ramp  slope=1/st  start=t  InitialOutput=0
  Saturation1 : Saturate  UpperLimit=1  LowerLimit=0
  Step2 : Step  Time=t  SampleTime=0
  Switch:kind1 : Switch  Criteria=u2 > Threshold  Threshold=0.5  SaturateOnIntegerOverflow=off  InputSameDT=off
  w_sim : Outport
  wires:
  RAMP1/1 -> Saturation1/1
  Saturation1/1 -> Switch:kind1/1
  Switch:kind1/1 -> Product1/2
  w/1 -> Product1/1
  Step2/1 -> Switch:kind1/3
  Product1/1 -> w_sim/1
  IncipF/1 -> Switch:kind1/2

== system TTS2_EXT/Faults/f-control1/calc_f9/Subsystem ==
  IncipF : Inport
  w : Inport  Port=2
  Product1 : Product
  RAMP1 : simulink/Sources/Ramp  slope=1/st  start=t  InitialOutput=0
  Saturation1 : Saturate  UpperLimit=1  LowerLimit=0
  Step2 : Step  Time=t  SampleTime=0
  Switch:kind1 : Switch  Criteria=u2 > Threshold  Threshold=0.5  SaturateOnIntegerOverflow=off  InputSameDT=off
  w_sim : Outport
  wires:
  RAMP1/1 -> Saturation1/1
  Saturation1/1 -> Switch:kind1/1
  Switch:kind1/1 -> Product1/2
  w/1 -> Product1/1
  Step2/1 -> Switch:kind1/3
  Product1/1 -> w_sim/1
  IncipF/1 -> Switch:kind1/2

== system TTS2_EXT/TTS2/Disturbance: Pump+pipe+control valve/VB/Positioner ==
  CV[0-100] : Inport
  Gain : Gain  Gain=0.01
  inertia : TransferFcn  Denominator=[0.1 1]
  X[0-1] : Outport  VectorParamsAs1DForOutWhenUnconnected=off
  wires:
  CV[0-100]/1 -> Gain/1
  Gain/1 -> inertia/1
  inertia/1 -> X[0-1]/1

== system TTS2_EXT/TTS2/Disturbance: Pump+pipe+control valve/VB/Valve ==
  G[0-1] : Inport
  P1[kPa] : Inport  Port=2
  P2[kPa] : Inport  Port=3
  Abs : Abs  SaturateOnIntegerOverflow=off
  Bus Creator : BusCreator  Inputs=4
  Product : Product
  Saturation : Saturate  UpperLimit=1  LowerLimit=0
  Sign : Signum
  Sum : Sum  Inputs=|+-
  Sum1 : Sum  Inputs=|+-
  Switch : Switch  Criteria=u2 > Threshold  SaturateOnIntegerOverflow=off  InputSameDT=off
  Transfer Fcn : TransferFcn  Denominator=[1 1]
  alfa : Constant
  kv_max : Constant  Value=0.000075
  lin_range : Constant
  liniowa : Subsystem
  ro : Constant
  stałoproc. : Subsystem
  F[m3/h] : Outport  VectorParamsAs1DForOutWhenUnconnected=off
  wires:
  G[0-1]/1 -> Saturation/1
  Saturation/1 -> liniowa/1(CV), stałoproc./1(CV), Sum/1
  P1[kPa]/1 -> Sum1/1
  P2[kPa]/1 -> Sum1/2
  Sum1/1 -> Sign/1, Abs/1
  kv_max/1 -> Bus Creator/1
  alfa/1 -> Bus Creator/2
  lin_range/1 -> Bus Creator/4, Sum/2
  ro/1 -> Bus Creator/3
  Switch/1 -> Product/1
  Product/1 -> Transfer Fcn/1
  Transfer Fcn/1 -> F[m3/h]/1
  Bus Creator/1 -> liniowa/3(param), stałoproc./3(param)
  Abs/1 -> liniowa/2(dP), stałoproc./2(dP)
  Sum/1 -> Switch/2
  Sign/1 -> Product/2
  stałoproc./1(F) -> Switch/1
  liniowa/1(F) -> Switch/3

== system TTS2_EXT/TTS2/Pump+pipe+control valve/V1/Positioner ==
  CV[0-100] : Inport
  Gain : Gain  Gain=0.01
  Saturation : Saturate  UpperLimit=1  LowerLimit=0
  inertia : TransferFcn  Denominator=[0.1 1]
  X[0-1] : Outport  VectorParamsAs1DForOutWhenUnconnected=off
  wires:
  CV[0-100]/1 -> Gain/1
  Gain/1 -> inertia/1
  inertia/1 -> Saturation/1
  Saturation/1 -> X[0-1]/1

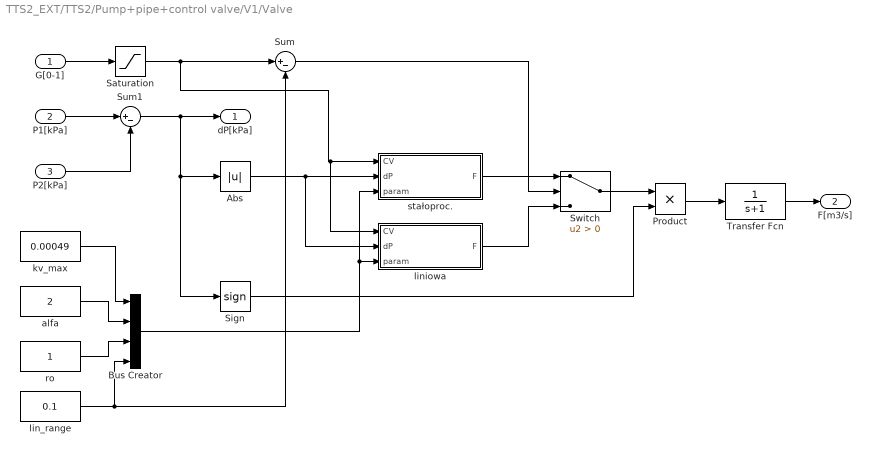
== system TTS2_EXT/TTS2/Pump+pipe+control valve/V1/Valve ==
  G[0-1] : Inport
  P1[kPa] : Inport  Port=2
  P2[kPa] : Inport  Port=3
  Abs : Abs  SaturateOnIntegerOverflow=off
  Bus Creator : BusCreator  Inputs=4
  Product : Product
  Saturation : Saturate  UpperLimit=1  LowerLimit=0
  Sign : Signum
  Sum : Sum  Inputs=|+-
  Sum1 : Sum  Inputs=|+-
  Switch : Switch  Criteria=u2 > Threshold  SaturateOnIntegerOverflow=off  InputSameDT=off
  Transfer Fcn : TransferFcn  Denominator=[1 1]
  alfa : Constant  Value=2
  kv_max : Constant  Value=0.00049
  lin_range : Constant  Value=0.1
  liniowa : Subsystem
  ro : Constant
  stałoproc. : Subsystem
  dP[kPa] : Outport  VectorParamsAs1DForOutWhenUnconnected=off
  F[m3/s] : Outport  Port=2  VectorParamsAs1DForOutWhenUnconnected=off
  wires:
  G[0-1]/1 -> Saturation/1
  Saturation/1 -> liniowa/1(CV), stałoproc./1(CV), Sum/1
  P1[kPa]/1 -> Sum1/1
  P2[kPa]/1 -> Sum1/2
  Sum1/1 -> dP[kPa]/1, Sign/1, Abs/1
  kv_max/1 -> Bus Creator/1
  alfa/1 -> Bus Creator/2
  lin_range/1 -> Bus Creator/4, Sum/2
  ro/1 -> Bus Creator/3
  Switch/1 -> Product/1
  Product/1 -> Transfer Fcn/1
  Transfer Fcn/1 -> F[m3/s]/1
  Bus Creator/1 -> liniowa/3(param), stałoproc./3(param)
  Abs/1 -> liniowa/2(dP), stałoproc./2(dP)
  Sum/1 -> Switch/2
  Sign/1 -> Product/2
  stałoproc./1(F) -> Switch/1
  liniowa/1(F) -> Switch/3

== system TTS2_EXT/TTS2/Pump+pipe+control valve/V1/f4 fault ==
  X : Inport
  str. : Inport  Port=2
  Add : Sum
  Fcn : Fcn  Expr=u(1)*((u(2)/100)+1)
  Manual Switch : ManualSwitch  CurrentSetting=0
  Mux : Mux  Inputs=2
  Xf : Outport  VectorParamsAs1DForOutWhenUnconnected=off
  wires:
  Mux/1 -> Fcn/1
  X/1 -> Add/1, Mux/1
  str./1 -> Add/2, Mux/2
  Add/1 -> Manual Switch/1
  Fcn/1 -> Manual Switch/2
  Manual Switch/1 -> Xf/1

== system TTS2_EXT/TTS2/Pump+pipe+control valve/V1/f6 fault ==
  X : Inport
  str. : Inport  Port=2
  Add : Sum
  Fcn : Fcn  Expr=u(1)*((u(2)/100)+1)
  Manual Switch : ManualSwitch  CurrentSetting=0
  Mux : Mux  Inputs=2
  Xf : Outport  VectorParamsAs1DForOutWhenUnconnected=off
  wires:
  Mux/1 -> Fcn/1
  X/1 -> Add/1, Mux/1
  str./1 -> Add/2, Mux/2
  Add/1 -> Manual Switch/1
  Fcn/1 -> Manual Switch/2
  Manual Switch/1 -> Xf/1

== system TTS2_EXT/TTS2/Pump+pipe+control valve/V2/Positioner ==
  CV[0-100] : Inport
  Gain : Gain  Gain=0.01
  Saturation : Saturate  UpperLimit=1  LowerLimit=0
  inertia : TransferFcn  Denominator=[0.1 1]
  X[0-1] : Outport  VectorParamsAs1DForOutWhenUnconnected=off
  wires:
  CV[0-100]/1 -> Gain/1
  Gain/1 -> inertia/1
  inertia/1 -> Saturation/1
  Saturation/1 -> X[0-1]/1

== system TTS2_EXT/TTS2/Pump+pipe+control valve/V2/Valve ==
  G[0-1] : Inport
  P1[kPa] : Inport  Port=2
  P2[kPa] : Inport  Port=3
  Abs : Abs  SaturateOnIntegerOverflow=off
  Bus Creator : BusCreator  Inputs=4
  Product : Product
  Saturation : Saturate  UpperLimit=1  LowerLimit=0
  Sign : Signum
  Sum : Sum  Inputs=|+-
  Sum1 : Sum  Inputs=|+-
  Switch : Switch  Criteria=u2 > Threshold  SaturateOnIntegerOverflow=off  InputSameDT=off
  Transfer Fcn : TransferFcn  Denominator=[1 1]
  alfa : Constant  Value=2
  kv_max : Constant  Value=0.00049
  lin_range : Constant  Value=0.1
  liniowa : Subsystem
  ro : Constant
  stałoproc. : Subsystem
  dP[kPa] : Outport  VectorParamsAs1DForOutWhenUnconnected=off
  F[m3/s] : Outport  Port=2  VectorParamsAs1DForOutWhenUnconnected=off
  wires:
  G[0-1]/1 -> Saturation/1
  Saturation/1 -> liniowa/1(CV), stałoproc./1(CV), Sum/1
  P1[kPa]/1 -> Sum1/1
  P2[kPa]/1 -> Sum1/2
  Sum1/1 -> dP[kPa]/1, Sign/1, Abs/1
  kv_max/1 -> Bus Creator/1
  alfa/1 -> Bus Creator/2
  lin_range/1 -> Bus Creator/4, Sum/2
  ro/1 -> Bus Creator/3
  Switch/1 -> Product/1
  Product/1 -> Transfer Fcn/1
  Transfer Fcn/1 -> F[m3/s]/1
  Bus Creator/1 -> liniowa/3(param), stałoproc./3(param)
  Abs/1 -> liniowa/2(dP), stałoproc./2(dP)
  Sum/1 -> Switch/2
  Sign/1 -> Product/2
  stałoproc./1(F) -> Switch/1
  liniowa/1(F) -> Switch/3

== system TTS2_EXT/TTS2/Pump+pipe+control valve/V2/f53 fault ==
  X : Inport
  str. : Inport  Port=2
  Add : Sum
  Fcn : Fcn  Expr=u(1)*((u(2)/100)+1)
  Manual Switch : ManualSwitch
  Mux : Mux  Inputs=2
  Xf : Outport  VectorParamsAs1DForOutWhenUnconnected=off
  wires:
  Mux/1 -> Fcn/1
  X/1 -> Add/1, Mux/1
  str./1 -> Add/2, Mux/2
  Add/1 -> Manual Switch/1
  Fcn/1 -> Manual Switch/2
  Manual Switch/1 -> Xf/1

== system TTS2_EXT/TTS2/Disturbance: Pump+pipe+control valve/VB/Valve/liniowa ==
  CV : Inport
  dP : Inport  Port=2
  param : Inport  Port=3
  Bus Selector : BusSelector  OutputSignals=signal4,signal2,signal1,signal3
  Fcn : Fcn  Expr=u(2)*(u(1)-1)
  Fcn1 : Fcn  Expr=sqrt(u(1)/u(2))/10
  Math Function : Math  SignedPower=on
  Mux : Mux  Inputs=2
  Mux1 : Mux  Inputs=2
  Product : Product  Inputs=*/***
  F : Outport  VectorParamsAs1DForOutWhenUnconnected=off
  wires:
  param/1 -> Bus Selector/1
  Fcn/1 -> Math Function/1
  Math Function/1 -> Product/1
  Product/1 -> F/1
  Mux/1 -> Fcn/1
  Mux1/1 -> Fcn1/1
  dP/1 -> Mux1/1
  Bus Selector/2 -> Mux/2  "<signal2>"
  Bus Selector/3 -> Product/3  "<signal1>"
  Fcn1/1 -> Product/5
  Bus Selector/4 -> Mux1/2  "<signal3>"
  Bus Selector/1 -> Product/2, Mux/1  "<signal4>"
  CV/1 -> Product/4

== system TTS2_EXT/TTS2/Disturbance: Pump+pipe+control valve/VB/Valve/stałoproc. ==
  CV : Inport
  dP : Inport  Port=2
  param : Inport  Port=3
  Bus Selector : BusSelector  OutputSignals=signal2,signal1,signal3
  Fcn : Fcn  Expr=u(2)*(u(1)-1)
  Fcn1 : Fcn  Expr=sqrt(u(1)/u(2))/10
  Math Function : Math  SignedPower=on
  Mux : Mux  Inputs=2
  Mux1 : Mux  Inputs=2
  Product : Product  Inputs=3
  F : Outport  VectorParamsAs1DForOutWhenUnconnected=off
  wires:
  param/1 -> Bus Selector/1
  Fcn/1 -> Math Function/1
  Math Function/1 -> Product/1
  Product/1 -> F/1
  CV/1 -> Mux/1
  Mux/1 -> Fcn/1
  Mux1/1 -> Fcn1/1
  dP/1 -> Mux1/1
  Bus Selector/1 -> Mux/2  "<signal2>"
  Bus Selector/2 -> Product/2  "<signal1>"
  Fcn1/1 -> Product/3
  Bus Selector/3 -> Mux1/2  "<signal3>"

== system TTS2_EXT/TTS2/Pump+pipe+control valve/V1/Valve/liniowa ==
  CV : Inport
  dP : Inport  Port=2
  param : Inport  Port=3
  Bus Selector : BusSelector  OutputSignals=signal4,signal2,signal1,signal3
  Fcn : Fcn  Expr=u(2)*(u(1)-1)
  Fcn1 : Fcn  Expr=sqrt(u(1)/u(2))/10
  Math Function : Math  SignedPower=on
  Mux : Mux  Inputs=2
  Mux1 : Mux  Inputs=2
  Product : Product  Inputs=*/***
  F : Outport  VectorParamsAs1DForOutWhenUnconnected=off
  wires:
  param/1 -> Bus Selector/1
  Fcn/1 -> Math Function/1
  Math Function/1 -> Product/1
  Product/1 -> F/1
  Mux/1 -> Fcn/1
  Mux1/1 -> Fcn1/1
  dP/1 -> Mux1/1
  Bus Selector/2 -> Mux/2  "<signal2>"
  Bus Selector/3 -> Product/3  "<signal1>"
  Fcn1/1 -> Product/5
  Bus Selector/4 -> Mux1/2  "<signal3>"
  Bus Selector/1 -> Product/2, Mux/1  "<signal4>"
  CV/1 -> Product/4

== system TTS2_EXT/TTS2/Pump+pipe+control valve/V1/Valve/stałoproc. ==
  CV : Inport
  dP : Inport  Port=2
  param : Inport  Port=3
  Bus Selector : BusSelector  OutputSignals=signal2,signal1,signal3
  Fcn : Fcn  Expr=u(2)*(u(1)-1)
  Fcn1 : Fcn  Expr=sqrt(u(1)/u(2))/10
  Math Function : Math  SignedPower=on
  Mux : Mux  Inputs=2
  Mux1 : Mux  Inputs=2
  Product : Product  Inputs=3
  F : Outport  VectorParamsAs1DForOutWhenUnconnected=off
  wires:
  param/1 -> Bus Selector/1
  Fcn/1 -> Math Function/1
  Math Function/1 -> Product/1
  Product/1 -> F/1
  CV/1 -> Mux/1
  Mux/1 -> Fcn/1
  Mux1/1 -> Fcn1/1
  dP/1 -> Mux1/1
  Bus Selector/1 -> Mux/2  "<signal2>"
  Bus Selector/2 -> Product/2  "<signal1>"
  Fcn1/1 -> Product/3
  Bus Selector/3 -> Mux1/2  "<signal3>"

== system TTS2_EXT/TTS2/Pump+pipe+control valve/V2/Valve/liniowa ==
  CV : Inport
  dP : Inport  Port=2
  param : Inport  Port=3
  Bus Selector : BusSelector  OutputSignals=signal4,signal2,signal1,signal3
  Fcn : Fcn  Expr=u(2)*(u(1)-1)
  Fcn1 : Fcn  Expr=sqrt(u(1)/u(2))/10
  Math Function : Math  SignedPower=on
  Mux : Mux  Inputs=2
  Mux1 : Mux  Inputs=2
  Product : Product  Inputs=*/***
  F : Outport  VectorParamsAs1DForOutWhenUnconnected=off
  wires:
  param/1 -> Bus Selector/1
  Fcn/1 -> Math Function/1
  Math Function/1 -> Product/1
  Product/1 -> F/1
  Mux/1 -> Fcn/1
  Mux1/1 -> Fcn1/1
  dP/1 -> Mux1/1
  Bus Selector/2 -> Mux/2  "<signal2>"
  Bus Selector/3 -> Product/3  "<signal1>"
  Fcn1/1 -> Product/5
  Bus Selector/4 -> Mux1/2  "<signal3>"
  Bus Selector/1 -> Product/2, Mux/1  "<signal4>"
  CV/1 -> Product/4

== system TTS2_EXT/TTS2/Pump+pipe+control valve/V2/Valve/stałoproc. ==
  CV : Inport
  dP : Inport  Port=2
  param : Inport  Port=3
  Bus Selector : BusSelector  OutputSignals=signal2,signal1,signal3
  Fcn : Fcn  Expr=u(2)*(u(1)-1)
  Fcn1 : Fcn  Expr=sqrt(u(1)/u(2))/10
  Math Function : Math  SignedPower=on
  Mux : Mux  Inputs=2
  Mux1 : Mux  Inputs=2
  Product : Product  Inputs=3
  F : Outport  VectorParamsAs1DForOutWhenUnconnected=off
  wires:
  param/1 -> Bus Selector/1
  Fcn/1 -> Math Function/1
  Math Function/1 -> Product/1
  Product/1 -> F/1
  CV/1 -> Mux/1
  Mux/1 -> Fcn/1
  Mux1/1 -> Fcn1/1
  dP/1 -> Mux1/1
  Bus Selector/1 -> Mux/2  "<signal2>"
  Bus Selector/2 -> Product/2  "<signal1>"
  Fcn1/1 -> Product/3
  Bus Selector/3 -> Mux1/2  "<signal3>"
